simulink model "VSGisland"  (R2015b)
settings: Solver=VariableStepAuto  StartTime=0.0  StopTime=1.0  RelTol=1e-3
undefined symbols (not defined in the file): plecs
libraries: powerlib x13, powerlib_extras x2, powerlib_meascontrol x1
settings Model: Creator=Administrator  LastModifiedBy=LXX

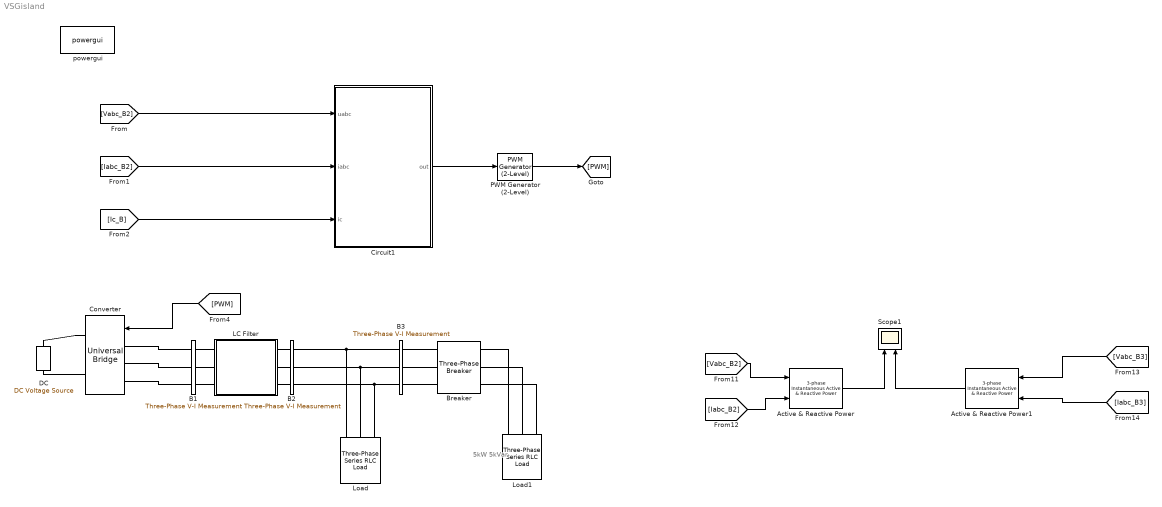
== system VSGisland ==
  note: 5kW
      | 5kVar
  Active & Reactive Power : powerlib_extras/Measurements/3-phase  Instantaneous  Active & Reactive Power
  Active & Reactive Power1 : powerlib_extras/Measurements/3-phase  Instantaneous  Active & Reactive Power
  B1 : powerlib/Measurements/Three-Phase V-I Measurement  VoltageMeasurement=phase-to-ground  SetLabelV=on  LabelV=Vabc_B1  Vpu=off  VpuLL=off  CurrentMeasurement=yes  SetLabelI=on  LabelI=Iabc_B1  Ipu=off  Pbase=100e6  Vbase=500e3  OutputType=Complex  PhasorSimulation=off  PSBequivalent=0
  B2 : powerlib/Measurements/Three-Phase V-I Measurement  VoltageMeasurement=phase-to-ground  SetLabelV=on  LabelV=Vabc_B2  Vpu=off  VpuLL=off  CurrentMeasurement=yes  SetLabelI=on  LabelI=Iabc_B2  Ipu=off  Pbase=100e6  Vbase=500e3  OutputType=Complex  PhasorSimulation=off  PSBequivalent=0
  B3 : powerlib/Measurements/Three-Phase V-I Measurement  VoltageMeasurement=phase-to-ground  SetLabelV=on  LabelV=Vabc_B3  Vpu=off  VpuLL=off  CurrentMeasurement=yes  SetLabelI=on  LabelI=Iabc_B3  Ipu=off  Pbase=100e6  Vbase=500e3  OutputType=Complex  PhasorSimulation=off  PSBequivalent=0
  Breaker : powerlib/Elements/Three-Phase Breaker  InitialState=open  SwitchA=on  SwitchB=on  SwitchC=on  SwitchTimes="[0.3  0.6]"  External=off  BreakerResistance=0.001  SnubberResistance=1e6  SnubberCapacitance=inf  Measurements=None
  Circuit1 : Subsystem  LoadFcn=plecs('sl', 200);  InitFcn=plecs('sl', 214);  StartFcn=plecs('sl', 208);  StopFcn=plecs('sl', 209);  mask(PlecsCircuit){PLECSData=<binary blob, 16808 chars, not shown>}
      mask prompts: PLECSData "PLECS Data (Do not delete or modify!)"
      mask init:
      | % PLACE CUSTOM INITIALIZATIONS ABOVE
      | % DO NOT REMOVE
      | plecs('sl', 215);
      | % DO NOT REMOVE
      settings: CopyFcn=plecs('sl', 203);  DeleteFcn=plecs('sl', 205);  UndoDeleteFcn=plecs('sl', 206);  PreSaveFcn=plecs('sl', 211);  PostSaveFcn=plecs('sl', 201);  NameChangeFcn=plecs('sl', 210);  DestroyFcn=plecs('sl', 207);  PreCopyFcn=plecs('sl', 216);  OpenFcn=plecs('sl', 202);  ErrorFcn=plerrorfcn
      mask Help: web(['file:///' fullfile(plecsdoc, 'creatingacircuit.html')])
      mask Display: disp('PLECS\nCircuit')
  Converter : powerlib/Power Electronics/Universal Bridge  Arms=3  SnubberResistance=1e5  SnubberCapacitance=inf  Device=IGBT / Diodes  Ron=1e-3  Lon=0  ForwardVoltages="[  0  0  ]"  ForwardVoltage=0  GTOparameters=[ 10e-6 , 20e-6 ]  IGBTparameters=[ 1e-6 , 2e-6 ]  Measurements=None  Measurements_2=None  converterType=Rectifier
  DC : powerlib/Electrical Sources/DC Voltage Source  Amplitude=800  Measurements=None
  LC Filter : Subsystem
  Load : powerlib/Elements/Three-Phase Series RLC Load  LConnTagsString=A|B|C  Configuration=Y (grounded)  NominalVoltage=380  Vabc=[1e3 1e3 1e3]  Vabcp=[1e3 1e3 1e3]  NominalFrequency=50  UnbalancedPower=off  ActivePower=10e3  InductivePower=10e3  CapacitivePower=0  Pabc=[10e3 9e3 11e3]  QLabc=[100 90 110]  QCabc=[100 90 110]  Pabcp=[10e3 9e3 11e3]  QLabcp=[100 90 110]  QCabcp=[100 90 110]  Measurements=None  LoadType=constant Z
  Load1 : powerlib/Elements/Three-Phase Series RLC Load  LConnTagsString=A|B|C  Configuration=Y (grounded)  NominalVoltage=380  Vabc=[1e3 1e3 1e3]  Vabcp=[1e3 1e3 1e3]  NominalFrequency=50  UnbalancedPower=off  ActivePower=5e3  InductivePower=5e3  CapacitivePower=0  Pabc=[10e3 9e3 11e3]  QLabc=[100 90 110]  QCabc=[100 90 110]  Pabcp=[10e3 9e3 11e3]  QLabcp=[100 90 110]  QCabcp=[100 90 110]  Measurements=None  LoadType=constant Z
  PWM Generator (2-Level) : powerlib_meascontrol/Pulse & Signal Generators/PWM Generator (2-Level)  ModulatorType=Three-phase bridge (6 pulses)  ModulatorMode=Unsynchronized  Fc=27*60  Pc=90  nF=27  MinMax="[ -1  1 ]"  SamplingTechnique=Natural  ModulatingSignals=off  m=0.8  Freq=60  Phase=0  Ts=0  ShowCarrierOutport=off
  Scope1 : Scope  NumInputPorts=2
  powergui : powerlib/powergui  Priority=1  SimulationMode=Discrete  SolverType=Tustin  SampleTime=5e-6  frequency=60  SPID=off  DisableSnubberDevices=off  DisableRonSwitches=off  DisableVfSwitches=off  SwTol=0  DisplayEquations=off  Interpol=off  ExternalGateDelay=off  methode=off  Ts=0  FunctionMessages=off  echomessages=off  HookPort=off  EnableUseOfTLC=off  x0status=blocks  frequencyindice=0  Pbase=100e6  ErrMax=1e-4  Iterations=50  UnitsV=kV  UnitsW=MW  buscounter=0  RestoreLinks=warning  ResistiveCurrentMeasurement=off  Frange=[0:2:500]  Ylog=off  Xlog=on  ShowGrid=off  save=off  variable=ZData  structure=0  ZoomFFT=off  StartTime=0.0  cycles=1  DisplayStyle=1  fundamental=60  FreqAxis=off  MaxFrequency=1000  frequencyindicesteady=1  RmsSteady=1  display=off
  wires:
  [PWM] -> Converter/1
  [Vabc_B2] -> Circuit1/1(uabc)
  [Iabc_B2] -> Circuit1/2(iabc)
  [Ic_B] -> Circuit1/3(ic)
  PWM Generator (2-Level)/1 -> [PWM]
  Circuit1/1(out) -> PWM Generator (2-Level)/1
  [Vabc_B2] -> Active & Reactive Power/1
  [Iabc_B2] -> Active & Reactive Power/2
  Active & Reactive Power/1 -> Scope1/1
  Active & Reactive Power1/1 -> Scope1/2
  [Vabc_B3] -> Active & Reactive Power1/1
  [Iabc_B3] -> Active & Reactive Power1/2
  connections:
  Converter/RConn1 -- DC/RConn1
  B1/RConn1 -- LC Filter/LConn1
  B1/RConn2 -- LC Filter/LConn2
  Converter/LConn1 -- B1/LConn1
  B2/LConn2 -- LC Filter/RConn2
  Converter/LConn3 -- B1/LConn3
  B2/LConn3 -- LC Filter/RConn3
  Converter/RConn2 -- DC/LConn1
  B2/LConn1 -- LC Filter/RConn1
  Converter/LConn2 -- B1/LConn2
  B1/RConn3 -- LC Filter/LConn3
  Load/LConn1 -- B2/RConn1 -- B3/LConn1
  Load/LConn2 -- B2/RConn2 -- B3/LConn2
  Load/LConn3 -- B2/RConn3 -- B3/LConn3
  Load1/LConn1 -- Breaker/RConn1
  Breaker/RConn3 -- Load1/LConn3
  B3/RConn2 -- Breaker/LConn2
  B3/RConn1 -- Breaker/LConn1
  B3/RConn3 -- Breaker/LConn3
  Breaker/RConn2 -- Load1/LConn2

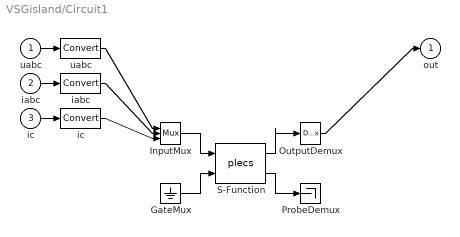
== system VSGisland/Circuit1 ==
  uabc : Inport  PortDimensions=3
  iabc : Inport  Port=2  PortDimensions=3
  ic : Inport  Port=3  PortDimensions=3
  " GateMux " : Ground
  " InputMux " : Mux  Inputs=[ 3 3 3 ]
  " OutputDemux " : Demux  Outputs=[ 3 ]
  " ProbeDemux " : Terminator
  " S-Function " : S-Function  FunctionName=plecs  SFunctionDeploymentMode=off  EnableBusSupport=off
  " iabc " : DataTypeConversion  SaturateOnIntegerOverflow=on  RndMeth=Zero
  " ic " : DataTypeConversion  SaturateOnIntegerOverflow=on  RndMeth=Zero
  " uabc " : DataTypeConversion  SaturateOnIntegerOverflow=on  RndMeth=Zero
  out : Outport  PortDimensions=3
  wires:
  " S-Function "/1 -> " OutputDemux "/1
  " InputMux "/1 -> " S-Function "/1
  " GateMux "/1 -> " S-Function "/2
  " S-Function "/2 -> " ProbeDemux "/1
  uabc/1 -> " uabc "/1
  " uabc "/1 -> " InputMux "/1
  iabc/1 -> " iabc "/1
  " iabc "/1 -> " InputMux "/2
  ic/1 -> " ic "/1
  " ic "/1 -> " InputMux "/3
  " OutputDemux "/1 -> out/1

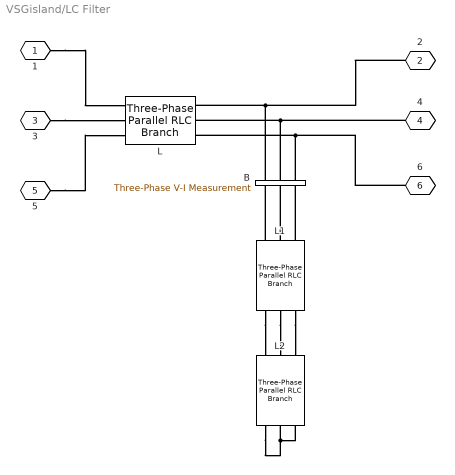
== system VSGisland/LC Filter ==
  B : powerlib/Measurements/Three-Phase V-I Measurement  VoltageMeasurement=phase-to-ground  SetLabelV=on  LabelV=Vc_B  Vpu=off  VpuLL=off  CurrentMeasurement=yes  SetLabelI=on  LabelI=Ic_B  Ipu=off  Pbase=100e6  Vbase=500e3  OutputType=Complex  PhasorSimulation=off  PSBequivalent=0
  L : powerlib/Elements/Three-Phase Parallel RLC Branch  LConnTagsString=A|B|C  RConnTagsString=A|B|C  BranchType=L  Resistance=1  Inductance=0.6e-3  Capacitance=1e-6  Measurements=None
  L1 : powerlib/Elements/Three-Phase Parallel RLC Branch  LConnTagsString=A|B|C  RConnTagsString=A|B|C  BranchType=R  Resistance=0.001  Inductance=1e-3  Capacitance=1e-6  Measurements=None
  L2 : powerlib/Elements/Three-Phase Parallel RLC Branch  LConnTagsString=A|B|C  RConnTagsString=A|B|C  BranchType=C  Resistance=1  Inductance=1e-3  Capacitance=1500e-6  Measurements=None
  1 : PMIOPort  Tag=PMCPort  Port=1  Side=Left
  2 : PMIOPort  Tag=PMCPort  Port=2  Side=Right
  3 : PMIOPort  Tag=PMCPort  Port=3  Side=Left
  4 : PMIOPort  Tag=PMCPort  Port=4  Side=Right
  5 : PMIOPort  Tag=PMCPort  Port=5  Side=Left
  6 : PMIOPort  Tag=PMCPort  Port=6  Side=Right
  connections:
  L1/RConn1 -- L2/LConn1
  L1/RConn2 -- L2/LConn2
  L1/RConn3 -- L2/LConn3
  B/LConn1 -- L/RConn1 -- 2/RConn1
  B/LConn2 -- L/RConn2 -- 4/RConn1
  B/LConn3 -- L/RConn3 -- 6/RConn1
  L2/RConn2 -- L2/RConn1 -- L2/RConn3
  L1/LConn1 -- B/RConn1
  L1/LConn2 -- B/RConn2
  L1/LConn3 -- B/RConn3
  1/RConn1 -- L/LConn1
  3/RConn1 -- L/LConn2
  5/RConn1 -- L/LConn3
